simulink library "null_allocation_lib"  (R2018b)
settings: Solver=VariableStepAuto  StartTime=0.0  StopTime=10.0  RelTol=1e-3
undefined symbols (not defined in the file or in its folder): fswParams
libraries: null_allocator x1
settings Model: Creator=Nick's PC  LastModifiedBy=Nick's PC

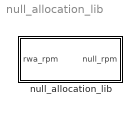
== system null_allocation_lib ==
  null_allocation_lib : Subsystem

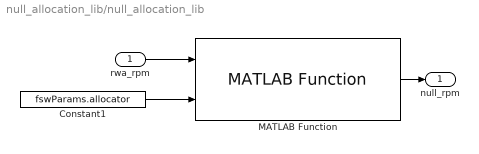
== system null_allocation_lib/null_allocation_lib ==
  rwa_rpm : Inport
  Constant1 : Constant  Value=fswParams.allocator  OutDataTypeStr=Bus: RWA
  MATLAB Function : null_allocator/MATLAB Function  SystemSampleTime=-1
  null_rpm : Outport
  wires:
  Constant1/1 -> MATLAB Function/2
  rwa_rpm/1 -> MATLAB Function/1
  MATLAB Function/1 -> null_rpm/1
